simulink model "DrvDem_CalcState"  (R2016b)
settings: configuration reference "CodeGenConfigSet" (kept outside this file)
values from neighbouring files (symbols this model uses):
  DrvDem_stShOffCfg_C = Calibration.Parameter    [init_DrvDem_CalcState.m]    (also in init_DrvDem_CalcState_SIL.m = Simulink.Parameter)
  DrvDem_tiNormal_C = Calibration.Parameter    [init_DrvDem_CalcState.m]    (also in init_DrvDem_CalcState_SIL.m = Simulink.Parameter)
  DrvDem_vThres_C = Calibration.Parameter    [init_DrvDem_CalcState.m]    (also in init_DrvDem_CalcState_SIL.m = Simulink.Parameter)
libraries: simulink x15
settings Model: Creator=zhoutinglin  LastModifiedBy=xuxingpei
settings ConfigSetRef: SourceLocation=Base Workspace

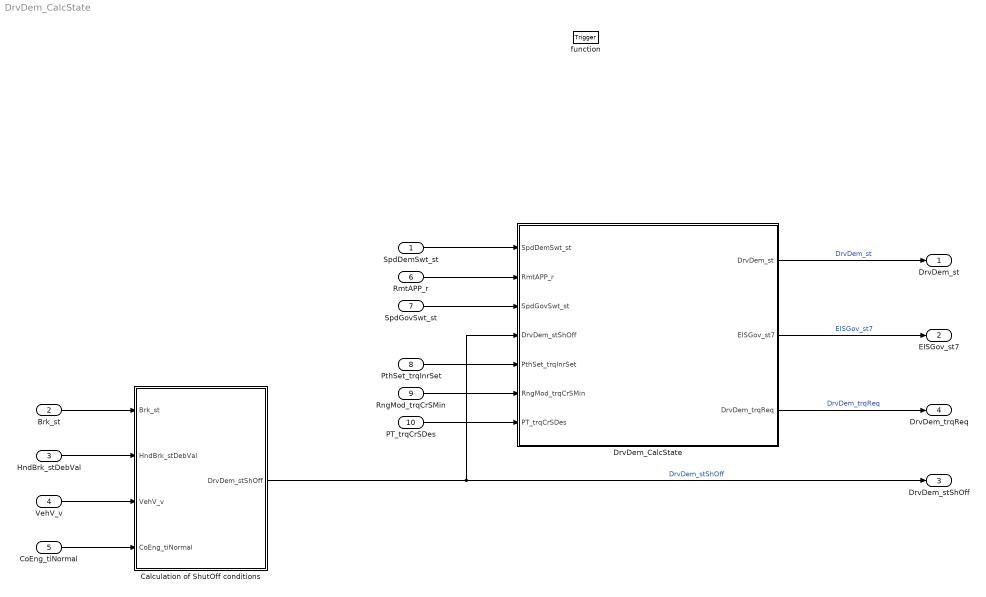
== system DrvDem_CalcState ==
  SpdDemSwt_st : Inport  Description=Speed demand switch status  OutMin=0  OutMax=1  OutDataTypeStr=boolean
  Brk_st : Inport  Description=Brake switch state  Port=2  OutMin=0  OutMax=255  OutDataTypeStr=State_uint8
  HndBrk_stDebVal : Inport  Description=Debounced value of Hand Brake switch  Port=3  OutMin=0  OutMax=255  OutDataTypeStr=State_uint8
  VehV_v : Inport  Tag=km/h  Description=Vehicle speed  Port=4  OutMin=0  OutMax=250  OutDataTypeStr=VehSpeed_km_h
  CoEng_tiNormal : Inport  Tag=ms  Description="Time since state\"CONENG_RUNNING\"was reached"  Port=5  OutMin=0  OutMax=42949672950  OutDataTypeStr=EngTime_ms
  RmtAPP_r : Inport  Tag=%  Description=Value of Remote accelerator pedal Position  Port=6  OutMin=0  OutMax=100  OutDataTypeStr=Accpedal_rate
  SpdGovSwt_st : Inport  Description=Speed Governor Switch status  Port=7  OutMin=0  OutMax=1  OutDataTypeStr=boolean
  PthSet_trqInrSet : Inport  Tag=Nm  Description=Inner torque set value after monitoring limitation  Port=8  OutMin=-3000  OutMax=3276.7  OutDataTypeStr=Trq_Nm
  RngMod_trqCrSMin : Inport  Tag=Nm  Description=minimal crankshaft torque  Port=9  OutMin=-3276.8  OutMax=3276.7  OutDataTypeStr=Trq_Nm
  PT_trqCrSDes : Inport  Tag=Nm  Description=Application parameter for requested propulsion torque to engine(crankshaft torque)  Port=10  OutMin=-3000  OutMax=3000  OutDataTypeStr=Trq_Nm
  function : TriggerPort  TriggerType=function-call  VariantControl=Variant
  Calculation of ShutOff conditions : Subsystem
  DrvDem_CalcState : Subsystem
  DrvDem_st : Outport  Description=Drive demand status to select the pedal for setpoint calculation  OutMin=0  OutMax=255  OutDataTypeStr=State_uint8
  EISGov_st7 : Outport  Description=Status information of DrvDem client  Port=2  OutMin=0  OutMax=2147483648  OutDataTypeStr=State_uint32
  DrvDem_stShOff : Outport  Description=ShutOff conditions from DrvDem  Port=3  OutMin=0  OutMax=255  OutDataTypeStr=State_uint8
  DrvDem_trqReq : Outport  Tag=Nm  Description=Requested initialisation torque to engine speed governor from DrvDem (with reference to the output)  Port=4  OutMin=-3000  OutMax=3000  OutDataTypeStr=Trq_Nm
  wires:
  DrvDem_CalcState/1(DrvDem_st) -> DrvDem_st/1  "DrvDem_st"
  DrvDem_CalcState/2(EISGov_st7) -> EISGov_st7/1  "EISGov_st7"
  SpdDemSwt_st/1 -> DrvDem_CalcState/1(SpdDemSwt_st)
  RmtAPP_r/1 -> DrvDem_CalcState/2(RmtAPP_r)
  Brk_st/1 -> Calculation of ShutOff conditions/1(Brk_st)
  HndBrk_stDebVal/1 -> Calculation of ShutOff conditions/2(HndBrk_stDebVal)
  VehV_v/1 -> Calculation of ShutOff conditions/3(VehV_v)
  CoEng_tiNormal/1 -> Calculation of ShutOff conditions/4(CoEng_tiNormal)
  Calculation of ShutOff conditions/1(DrvDem_stShOff) -> DrvDem_CalcState/4(DrvDem_stShOff), DrvDem_stShOff/1  "DrvDem_stShOff"
  SpdGovSwt_st/1 -> DrvDem_CalcState/3(SpdGovSwt_st)
  DrvDem_CalcState/3(DrvDem_trqReq) -> DrvDem_trqReq/1  "DrvDem_trqReq"
  PthSet_trqInrSet/1 -> DrvDem_CalcState/5(PthSet_trqInrSet)
  RngMod_trqCrSMin/1 -> DrvDem_CalcState/6(RngMod_trqCrSMin)
  PT_trqCrSDes/1 -> DrvDem_CalcState/7(PT_trqCrSDes)

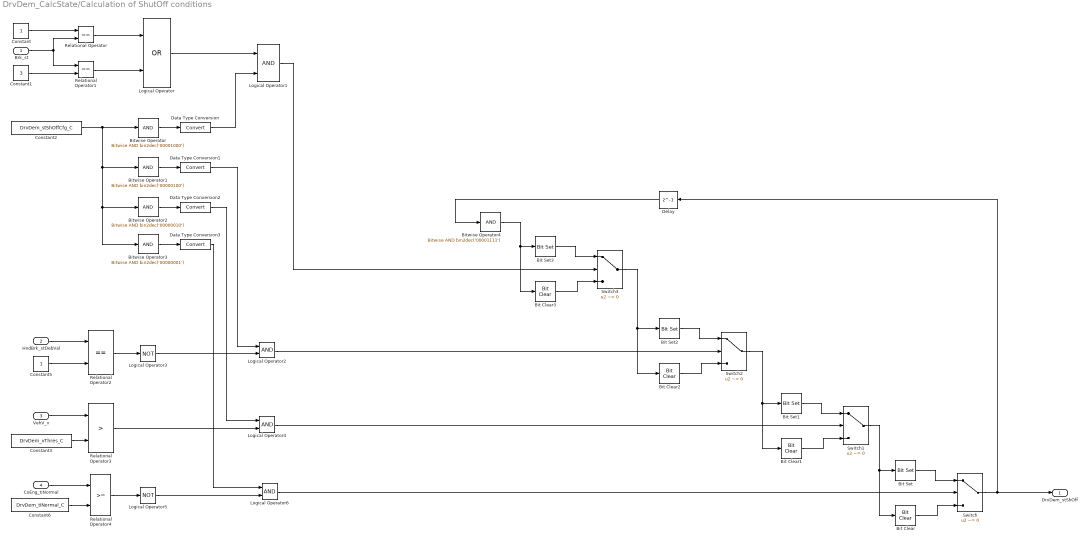
== system DrvDem_CalcState/Calculation of ShutOff conditions ==
  Brk_st : Inport  Description=Brake switch state
  HndBrk_stDebVal : Inport  Description=Debounced value of Hand Brake switch  Port=2
  VehV_v : Inport  Tag=km/h  Description=Vehicle speed  Port=3
  CoEng_tiNormal : Inport  Tag=ms  Description="Time since state\"CONENG_RUNNING\"was reached"  Port=4
  Bit Clear : simulink/Logic and Bit Operations/Bit Clear  iBit=0
  Bit Clear1 : simulink/Logic and Bit Operations/Bit Clear  iBit=1
  Bit Clear2 : simulink/Logic and Bit Operations/Bit Clear  iBit=2
  Bit Clear3 : simulink/Logic and Bit Operations/Bit Clear  iBit=3
  Bit Set : simulink/Logic and Bit Operations/Bit Set  iBit=0
  Bit Set1 : simulink/Logic and Bit Operations/Bit Set  iBit=1
  Bit Set2 : simulink/Logic and Bit Operations/Bit Set  iBit=2
  Bit Set3 : simulink/Logic and Bit Operations/Bit Set  iBit=3
  Bitwise Operator : simulink/Logic and Bit Operations/Bitwise Operator  logicop=AND  UseBitMask=on  BitMask=bin2dec('00001000')  BitMaskRealWorld=Stored Integer
  Bitwise Operator1 : simulink/Logic and Bit Operations/Bitwise Operator  logicop=AND  UseBitMask=on  BitMask=bin2dec('00000100')  BitMaskRealWorld=Stored Integer
  Bitwise Operator2 : simulink/Logic and Bit Operations/Bitwise Operator  logicop=AND  UseBitMask=on  BitMask=bin2dec('00000010')  BitMaskRealWorld=Stored Integer
  Bitwise Operator3 : simulink/Logic and Bit Operations/Bitwise Operator  logicop=AND  UseBitMask=on  BitMask=bin2dec('00000001')  BitMaskRealWorld=Stored Integer
  Bitwise Operator4 : simulink/Logic and Bit Operations/Bitwise Operator  logicop=AND  UseBitMask=on  BitMask=bin2dec('00001111')  BitMaskRealWorld=Stored Integer
  Constant : Constant  OutDataTypeStr=Inherit: Inherit via back propagation
  Constant1 : Constant  Value=3  OutDataTypeStr=Inherit: Inherit via back propagation
  Constant2 : Constant  Value=DrvDem_stShOffCfg_C
  Constant3 : Constant  Value=DrvDem_vThres_C
  Constant5 : Constant  OutDataTypeStr=Inherit: Inherit via back propagation
  Constant6 : Constant  Value=DrvDem_tiNormal_C
  Data Type Conversion{,1..3} (4 alike) : DataTypeConversion
  Delay : Delay  DelayLength=1  InitialCondition=0
  Logical Operator : Logic  Operator=OR  AllPortsSameDT=off  OutDataTypeStr=boolean
  Logical Operator{1..2,4,6} (4 alike) : Logic  AllPortsSameDT=off  OutDataTypeStr=boolean
  Logical Operator3 : Logic  Operator=NOT  AllPortsSameDT=off  OutDataTypeStr=boolean
  Logical Operator5 : Logic  Operator=NOT  AllPortsSameDT=off  OutDataTypeStr=boolean
  Relational Operator : RelationalOperator  Operator===  OutDataTypeStr=boolean  RndMeth=Simplest  InputSameDT=on
  Relational Operator1 : RelationalOperator  Operator===  OutDataTypeStr=boolean  RndMeth=Simplest  InputSameDT=on
  Relational Operator2 : RelationalOperator  Operator===  OutDataTypeStr=boolean  RndMeth=Simplest  InputSameDT=on
  Relational Operator3 : RelationalOperator  Operator=>  OutDataTypeStr=boolean  RndMeth=Simplest
  Relational Operator4 : RelationalOperator  OutDataTypeStr=boolean  RndMeth=Simplest
  Switch{,1..3} (4 alike) : Switch  Criteria=u2 ~= 0
  DrvDem_stShOff : Outport  Description=ShutOff conditions from DrvDem
  wires:
  Constant/1 -> Relational Operator/1
  Brk_st/1 -> Relational Operator1/1, Relational Operator/2
  Constant1/1 -> Relational Operator1/2
  Relational Operator/1 -> Logical Operator/1
  Relational Operator1/1 -> Logical Operator/2
  Constant2/1 -> Bitwise Operator3/1, Bitwise Operator2/1, Bitwise Operator1/1, Bitwise Operator/1
  HndBrk_stDebVal/1 -> Relational Operator2/1
  Constant5/1 -> Relational Operator2/2
  Logical Operator/1 -> Logical Operator1/1
  Bitwise Operator/1 -> Data Type Conversion/1
  Bitwise Operator1/1 -> Data Type Conversion1/1
  Relational Operator2/1 -> Logical Operator3/1
  Logical Operator3/1 -> Logical Operator2/2
  VehV_v/1 -> Relational Operator3/1
  Constant3/1 -> Relational Operator3/2
  Relational Operator3/1 -> Logical Operator4/2
  Bitwise Operator2/1 -> Data Type Conversion2/1
  CoEng_tiNormal/1 -> Relational Operator4/1
  Constant6/1 -> Relational Operator4/2
  Relational Operator4/1 -> Logical Operator5/1
  Logical Operator5/1 -> Logical Operator6/2
  Bitwise Operator3/1 -> Data Type Conversion3/1
  Switch/1 -> Delay/1, DrvDem_stShOff/1
  Bit Set/1 -> Switch/1
  Bit Clear/1 -> Switch/3
  Logical Operator6/1 -> Switch/2
  Bit Set1/1 -> Switch1/1
  Bit Clear1/1 -> Switch1/3
  Switch1/1 -> Bit Clear/1, Bit Set/1
  Logical Operator4/1 -> Switch1/2
  Bit Set2/1 -> Switch2/1
  Bit Clear2/1 -> Switch2/3
  Switch2/1 -> Bit Set1/1, Bit Clear1/1
  Logical Operator2/1 -> Switch2/2
  Bit Set3/1 -> Switch3/1
  Bit Clear3/1 -> Switch3/3
  Switch3/1 -> Bit Set2/1, Bit Clear2/1
  Logical Operator1/1 -> Switch3/2
  Delay/1 -> Bitwise Operator4/1
  Bitwise Operator4/1 -> Bit Set3/1, Bit Clear3/1
  Data Type Conversion/1 -> Logical Operator1/2
  Data Type Conversion1/1 -> Logical Operator2/1
  Data Type Conversion2/1 -> Logical Operator4/1
  Data Type Conversion3/1 -> Logical Operator6/1

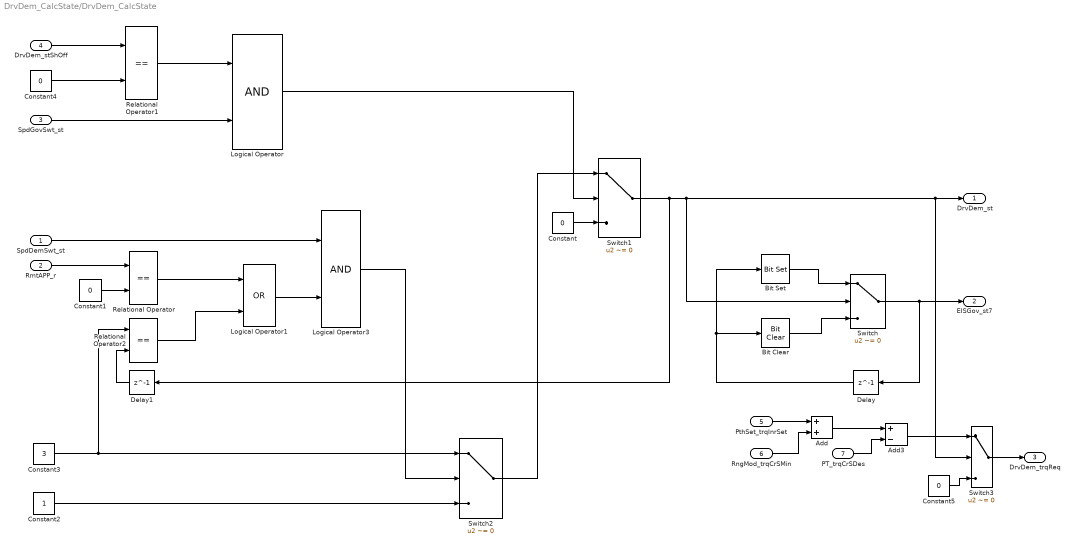
== system DrvDem_CalcState/DrvDem_CalcState ==
  SpdDemSwt_st : Inport  Description=Speed demand switch status
  RmtAPP_r : Inport  Description=Speed demand switch status  Port=2
  SpdGovSwt_st : Inport  Description=Speed Governor Switch status  Port=3
  DrvDem_stShOff : Inport  Description=Speed demand switch status  Port=4
  PthSet_trqInrSet : Inport  Tag=Nm  Description=Inner torque set value after monitoring limitation  Port=5
  RngMod_trqCrSMin : Inport  Port=6
  PT_trqCrSDes : Inport  Port=7
  Add : Sum  SaturateOnIntegerOverflow=on
  Add3 : Sum  Inputs=+-  SaturateOnIntegerOverflow=on
  Bit Clear : simulink/Logic and Bit Operations/Bit Clear  iBit=7
  Bit Set : simulink/Logic and Bit Operations/Bit Set  iBit=7
  Constant{,1,4..5} (4 alike) : Constant  Value=0  OutDataTypeStr=Inherit: Inherit via back propagation
  Constant2 : Constant  OutDataTypeStr=Inherit: Inherit via back propagation
  Constant3 : Constant  Value=3  OutDataTypeStr=Inherit: Inherit via back propagation
  Delay : Delay  DelayLength=1  InitialCondition=0
  Delay1 : Delay  DelayLength=1  InitialCondition=0
  Logical Operator : Logic  AllPortsSameDT=off  OutDataTypeStr=boolean
  Logical Operator1 : Logic  Operator=OR  AllPortsSameDT=off  OutDataTypeStr=boolean
  Logical Operator3 : Logic  AllPortsSameDT=off  OutDataTypeStr=boolean
  Relational Operator : RelationalOperator  Operator===  OutDataTypeStr=boolean  RndMeth=Simplest  InputSameDT=on
  Relational Operator1 : RelationalOperator  Operator===  OutDataTypeStr=boolean  RndMeth=Simplest  InputSameDT=on
  Relational Operator2 : RelationalOperator  Operator===  OutDataTypeStr=boolean  RndMeth=Simplest
  Switch : Switch  Criteria=u2 ~= 0
  Switch1 : Switch  Criteria=u2 ~= 0  InputSameDT=on
  Switch2 : Switch  Criteria=u2 ~= 0  InputSameDT=on
  Switch3 : Switch  Criteria=u2 ~= 0
  DrvDem_st : Outport  Description=Drive demand status to select the pedal for setpoint calculation
  EISGov_st7 : Outport  Description=Status information of DrvDem client  Port=2
  DrvDem_trqReq : Outport  Tag=Nm  Description=Requested initialisation torque to engine speed governor from DrvDem (with reference to the output)  Port=3
  wires:
  Switch/1 -> Delay/1, EISGov_st7/1
  Bit Set/1 -> Switch/1
  Bit Clear/1 -> Switch/3
  Delay/1 -> Bit Set/1, Bit Clear/1
  Switch1/1 -> Delay1/1, Switch3/2, DrvDem_st/1, Switch/2
  Constant/1 -> Switch1/3
  RmtAPP_r/1 -> Relational Operator/1
  Constant1/1 -> Relational Operator/2
  DrvDem_stShOff/1 -> Relational Operator1/1
  Constant4/1 -> Relational Operator1/2
  Relational Operator1/1 -> Logical Operator/1
  Logical Operator/1 -> Switch1/2
  Switch2/1 -> Switch1/1
  Constant2/1 -> Switch2/3
  Constant3/1 -> Relational Operator2/1, Switch2/1
  Relational Operator/1 -> Logical Operator1/1
  Relational Operator2/1 -> Logical Operator1/2
  Delay1/1 -> Relational Operator2/2
  Logical Operator1/1 -> Logical Operator3/2
  Logical Operator3/1 -> Switch2/2
  SpdGovSwt_st/1 -> Logical Operator/2
  SpdDemSwt_st/1 -> Logical Operator3/1
  PthSet_trqInrSet/1 -> Add/1
  RngMod_trqCrSMin/1 -> Add/2
  Add/1 -> Add3/1
  PT_trqCrSDes/1 -> Add3/2
  Add3/1 -> Switch3/1
  Switch3/1 -> DrvDem_trqReq/1
  Constant5/1 -> Switch3/3
